simulink model "nadrz_01"  (R2017a)
settings: Solver=ode45  StartTime=0.0  StopTime=300  FixedStep=0.01  MaxStep=0.2  RelTol=1e-3  EnableMultiTasking=on
libraries: fuzblock x1
settings Model: Creator=Administrator  LastModifiedBy=pouzivatel
settings DataIOCC: LimitDataPoints=on  SaveFormat=Array  SignalLoggingSaveFormat=ModelDataLogs  SignalLoggingName=sigsOut
settings OptimizationCC: BooleanDataType=off  ExpressionDepthLimit=2147483647  InitFltsAndDblsToZero=on  LifeSpan=inf
settings DebuggingCC: SaveWithParameterizedLinksMsg=none  UnderspecifiedInitializationDetection=Classic  MergeDetectMultiDrivingBlocksExec=none  SignalResolutionControl=TryResolveAllWithWarning  MultiTaskDSMMsg=warning  MultiTaskCondExecSysMsg=none  FcnCallInpInsideContextMsg=warning  StateNameClashWarn=warning  SFUnexpectedBacktrackingDiag=warning  SFNoUnconditionalDefaultTransitionDiag=warning  SFExecutionAtInitializationDiag=none
settings HardwareCC: ProdBitPerPointer=32  ProdBitPerSizeT=32  ProdBitPerPtrDiffT=32  ProdLargestAtomicFloat=None  ProdIntDivRoundTo=Undefined  ProdEndianess=Unspecified  ProdWordSize=32  ProdHWDeviceType=32-bit Generic  TargetUnknown=on
settings ModelReferenceCC: PropagateSignalLabelsOutOfModel=off
settings GRTTargetCC: TargetFcnLib=ansi_tfl_tmw.mat  TargetLangStandard=C89/C90 (ANSI)  CombineOutputUpdateFcns=off  GRTInterface=on
settings ConfigComp: CovMetricSettings=dw  CovHtmlReporting=on  CovSaveCumulativeToWorkspaceVar=on  CovSaveSingleToWorkspaceVar=on  CovExternalEMLEnable=off

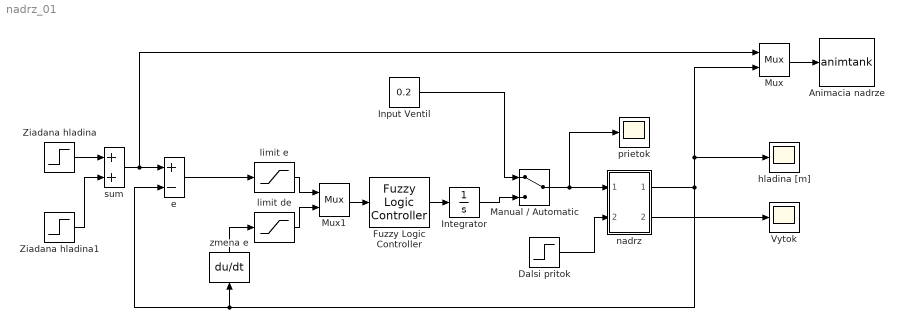
== system nadrz_01 ==
  Animacia nadrze : S-Function  FunctionName=animtank  Parameters=1  SFunctionDeploymentMode=off  EnableBusSupport=off
  Dalsi pritok : Step  Time=200  After=0.1  SampleTime=0
  Fuzzy Logic Controller : fuzblock/Fuzzy Logic  Controller  fis=fuzreg02
  Input Ventil : Constant  Value=0.2
  Integrator : Integrator  LimitOutput=on  UpperSaturationLimit=0.3  LowerSaturationLimit=0
  Manual / Automatic : ManualSwitch
  Mux : Mux  Inputs=2
  Mux1 : Mux  Inputs=2
  "Vytok " : Scope
  Ziadana hladina : Step  Time=5  After=1.001  SampleTime=0
  Ziadana hladina1 : Step  Time=100  After=-0.5  SampleTime=0
  e : Sum  Inputs=+-  SaturateOnIntegerOverflow=on  InputSameDT=on  OutDataTypeStr=Inherit: Same as first input
  hladina [m] : Scope
  limit de : Saturate  UpperLimit=0.3  LowerLimit=-0.3
  limit e : Saturate  UpperLimit=2  LowerLimit=-2
  nadrz : Subsystem
  prietok : Scope
  sum : Sum  SaturateOnIntegerOverflow=on  InputSameDT=on  OutDataTypeStr=Inherit: Same as first input
  zmena e : Derivative
  wires:
  Mux/1 -> Animacia nadrze/1
  nadrz/1(Out1) -> hladina [m]/1, Mux/2, e/2, zmena e/1
  Manual / Automatic/1 -> nadrz/1(In1), prietok/1
  Fuzzy Logic Controller/1 -> Integrator/1
  e/1 -> limit e/1
  Dalsi pritok/1 -> nadrz/2(In2)
  nadrz/2(Out2) -> "Vytok "/1
  Input Ventil/1 -> Manual / Automatic/1
  Ziadana hladina/1 -> sum/1
  Ziadana hladina1/1 -> sum/2
  sum/1 -> e/1, Mux/1
  zmena e/1 -> limit de/1
  limit de/1 -> Mux1/2
  limit e/1 -> Mux1/1
  Mux1/1 -> Fuzzy Logic Controller/1
  Integrator/1 -> Manual / Automatic/2

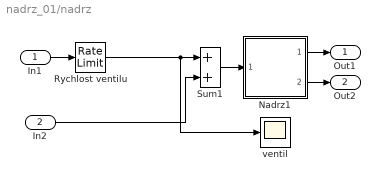
== system nadrz_01/nadrz ==
  In1 : Inport
  In2 : Inport  Port=2
  Nadrz1 : Subsystem  mask(Water tank){ht=2, area=1, outletArea=0.05, overflowLimit=0, initialHt=0}
      mask prompts: ht "Height of tank (m):"; area "Bottom area (m^2):"; outletArea "Out pipe crossection (m^2):"; overflowLimit "Overflow sensor distance from top (m):"; initialHt "Initial level height (m):"
      mask help: Cylindrical water tank with overflow signal
      mask Display: disp('WATER\nTANK')
  Rychlost ventilu : RateLimiter  RisingSlewLimit=0.015  FallingSlewLimit=-0.015
  Sum1 : Sum  SaturateOnIntegerOverflow=on  InputSameDT=on  OutDataTypeStr=Inherit: Same as first input
  ventil : Scope
  Out1 : Outport
  Out2 : Outport  Port=2
  wires:
  Rychlost ventilu/1 -> Sum1/1, ventil/1
  Nadrz1/1(water level) -> Out1/1
  In1/1 -> Rychlost ventilu/1
  In2/1 -> Sum1/2
  Nadrz1/2(flow out) -> Out2/1
  Sum1/1 -> Nadrz1/1(flow in)

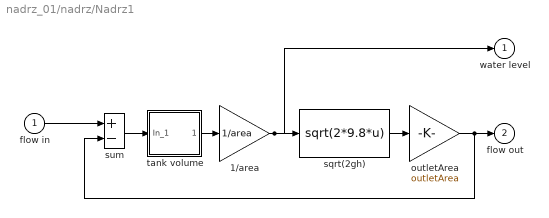
== system nadrz_01/nadrz/Nadrz1 ==
  flow in : Inport
  1/area : Gain  Gain=1/area  SaturateOnIntegerOverflow=on  OutDataTypeStr=Inherit: Same as input  ParamDataTypeStr=Inherit: Same as input
  outletArea : Gain  Gain=outletArea  SaturateOnIntegerOverflow=on  OutDataTypeStr=Inherit: Same as input  ParamDataTypeStr=Inherit: Same as input
  sqrt(2gh) : Fcn  Expr=sqrt(2*9.8*u)
  sum : Sum  Inputs=+-  SaturateOnIntegerOverflow=on  InputSameDT=on  OutDataTypeStr=Inherit: Same as first input
  tank volume : Subsystem  mask(Limited integrator.){lb=0, ub=ht * area, xi=0}
      mask prompts: lb "Lower bound:"; ub "Upper bound:"; xi "Initial condition"
      mask help: Limited integrator
      mask Help: Implements a limited integrator with \nan expression of the form:\n\nif(x<=lb and u<0) or (x>=ub and u>0)\n\txdot=0\nelse\n\txdot=u.
      mask Display: plot(-1,-0.2,3.5,1.2,[0.05,1,2,2.9],[0,0,1,1]);disp(' 1/s    ')
  water level : Outport  InitialOutput=0
  flow out : Outport  Port=2  InitialOutput=0
  wires:
  outletArea/1 -> flow out/1, sum/2
  sqrt(2gh)/1 -> outletArea/1
  1/area/1 -> water level/1, sqrt(2gh)/1
  tank volume/1(Out_1) -> 1/area/1
  flow in/1 -> sum/1
  sum/1 -> tank volume/1(In_1)

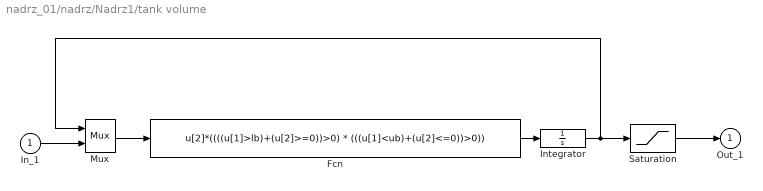
== system nadrz_01/nadrz/Nadrz1/tank volume ==
  In_1 : Inport
  Fcn : Fcn  Expr=u[2]*((((u[1]>lb)+(u[2]>=0))>0) * (((u[1]<ub)+(u[2]<=0))>0))
  Integrator : Integrator  InitialCondition=xi
  Mux : Mux  Inputs=2
  Saturation : Saturate  UpperLimit=ub  LowerLimit=lb
  Out_1 : Outport  InitialOutput=0
  wires:
  Integrator/1 -> Saturation/1, Mux/1
  Fcn/1 -> Integrator/1
  Mux/1 -> Fcn/1
  In_1/1 -> Mux/2
  Saturation/1 -> Out_1/1
